simulink model "snap2_f_200msps_64i_4096c"  (R2019a)
settings: Solver=VariableStepDiscrete  StartTime=0.0  StopTime=10.0  RelTol=1e-3
undefined symbols (not defined in the file or in its folder): datetime, posixtime
libraries: xbsIndex_r4 x21354, casper_library_misc x297, casper_library_delays x19, xps_library x14, casper_library_sources x4
(part 34 of 217)

== system snap2_f_200msps_64i_4096c/noise/octal_mux4 ==
  n0 : Inport
  n1 : Inport  Port=2
  n2 : Inport  Port=3
  n3 : Inport  Port=4
  Delay{,1..7} (8 alike) : xbsIndex_r4/Delay  rst=off  infoeditControl=Selection of Reset will increase slice count due to use of real FFs and instead of SRLs  en=off  latency=1  reg_retiming=off  dbl_ovrd=off  block_type=delay
  Mux{,1..7} (8 alike) : xbsIndex_r4/Mux  inputs=4  en=off  latency=1  precision=Full  arith_type=Unsigned  n_bits=16  bin_pt=14  quantization=Truncate  overflow=Wrap  dbl_ovrd=off  block_type=mux
  Slice{,1..7} (8 alike) : xbsIndex_r4/Slice  nbits=2  boolean_output=off  mode=Lower Bit Location + Width  bit1=0  base1=MSB of Input  bit0=0  base0=LSB of Input  dbl_ovrd=off  block_type=slice
  bus_expand : Subsystem  AncestorBlock=casper_library_flow_control/bus_expand  mask(bus_expand){mode=divisions of equal size, outputNum=8, outputWidth=4, outputBinaryPt=0, outputArithmeticType=0, show_format=off, outputToWorkspace=off, variablePrefix=out, outputToModelAsWell=on}
      mask prompts: outputNum "Number of outputs:"; outputWidth "Output width:"; outputBinaryPt "Output binary point position:"; outputArithmeticType "Output arithmetic type (ufix=0, fix=1, bool=2):"; show_format "Print format string?"; outputToWorkspace "Output to workspace?"; variablePrefix "Variable name prefix:"; outputToModelAsWell "Output to model as well?"
      mask help:
      | Expands a 'bus' made using a bus_create or Xilinx
      | concat block.
      | The input will be divided into the specified number
      | of outputs with the specified arithmetic types.
      | Divisions are made from most significant bit.
      mask init: same as snap2_f_200msps_64i_4096c/autocorr/bus_expand
      settings: AttributesFormatString=8 outputs
      mask TypeOptions mode: divisions of equal size | divisions of arbitrary size
      mask Callback mode: bus_expand_callback();
      mask Callback outputWidth: bus_expand_callback();
      mask Callback outputToWorkspace: bus_expand_callback();
  sel : Subsystem  Tag=xps:sw_reg  AncestorBlock=xps_library/Memory/software_register  mask(swreg){io_dir=From Processor, io_delay=0, init_val=0, sample_period=1, names=reg, bitwidths=32, bin_pts=0, arith_types=0, sim_port=on, show_format=on, desc_str=|}
      mask desc_str=|
      | The lower 2 bits define the select signal for the
      | noise multiplexor. If this register has value ``v``, then noise generator
      | ``v`` is selected.
      mask prompts: io_dir "I/O direction"; io_delay "I/O delay"; init_val "Initial Value"; sample_period "Sample period"; names "Bitfield names [msb...lsb]"; bitwidths "Bitfield widths"; bin_pts "Bitfield binary pts"; arith_types "Bitfield types, ufix=0, fix=1, bool=2"; sim_port "Provide sim input/output?"; show_format "Print format string?"; desc_str "Description"
      mask help: A 32-bit software-accessible register. Can be divided into bitfields of varying widths and types using the fields in the block mask.
      mask init:
      | swreg_init(gcb)
      settings: AttributesFormatString=1input:uf32.0 = 32 bits
      mask TypeOptions io_dir: To Processor | From Processor
      mask Callback io_dir:
      | mask_enables = get_param(gcb, 'MaskEnables');
      | mask_names = get_param(gcb, 'MaskNames');
      | if strcmp(get_param(gcb, 'io_dir'), 'To Processor'),
      |     mask_enables{ismember(mask_names, 'sample_period')} = 'off';
      | else
      |     mask_enables{ismember(mask_names, 'sample_period')} = 'on';
      | end
      | set_param(gcb, 'MaskEnables', mask_enables);
      mask DialogControl ParameterTabVar0 Prompt: Setup
  out0 : Outport
  out1 : Outport  Port=2
  out2 : Outport  Port=3
  out3 : Outport  Port=4
  out4 : Outport  Port=5
  out5 : Outport  Port=6
  out6 : Outport  Port=7
  out7 : Outport  Port=8
  wires:
  Mux/1 -> out0/1
  n0/1 -> [noise0]
  n1/1 -> [noise1]
  n2/1 -> [noise2]
  n3/1 -> [noise3]
  [sel0] -> Delay/1
  [noise0] -> Mux/2
  [noise1] -> Mux/3
  [noise2] -> Mux/4
  [noise3] -> Mux/5
  [sel1] -> Delay1/1
  Mux1/1 -> out1/1
  sel/1(in_reg) -> bus_expand/1(bus_in)
  bus_expand/8(lsb_out1) -> Slice7/1
  bus_expand/7(out2) -> Slice6/1
  bus_expand/1(msb_out8) -> Slice/1
  bus_expand/2(out7) -> Slice1/1
  bus_expand/3(out6) -> Slice2/1
  bus_expand/4(out5) -> Slice3/1
  bus_expand/5(out4) -> Slice4/1
  bus_expand/6(out3) -> Slice5/1
  Mux3/1 -> out3/1
  [sel3] -> Delay3/1
  [sel2] -> Delay2/1
  Mux2/1 -> out2/1
  Mux6/1 -> out6/1
  [sel6] -> Delay5/1
  [sel7] -> Delay4/1
  Mux7/1 -> out7/1
  Mux5/1 -> out5/1
  [sel5] -> Delay6/1
  [sel4] -> Delay7/1
  Mux4/1 -> out4/1
  Slice/1 -> [sel7]
  Slice1/1 -> [sel6]
  Slice2/1 -> [sel5]
  Slice3/1 -> [sel4]
  Slice4/1 -> [sel3]
  Slice5/1 -> [sel2]
  Slice6/1 -> [sel1]
  Slice7/1 -> [sel0]
  [noise3] -> Mux1/5
  [noise2] -> Mux1/4
  [noise1] -> Mux1/3
  [noise0] -> Mux1/2
  [noise0] -> Mux2/2
  [noise1] -> Mux2/3
  [noise2] -> Mux2/4
  [noise3] -> Mux2/5
  [noise3] -> Mux3/5
  [noise2] -> Mux3/4
  [noise1] -> Mux3/3
  [noise0] -> Mux3/2
  [noise0] -> Mux4/2
  [noise1] -> Mux4/3
  [noise2] -> Mux4/4
  [noise3] -> Mux4/5
  [noise3] -> Mux5/5
  [noise2] -> Mux5/4
  [noise1] -> Mux5/3
  [noise0] -> Mux5/2
  [noise0] -> Mux6/2
  [noise1] -> Mux6/3
  [noise2] -> Mux6/4
  [noise3] -> Mux6/5
  [noise3] -> Mux7/5
  [noise2] -> Mux7/4
  [noise1] -> Mux7/3
  [noise0] -> Mux7/2
  Delay/1 -> Mux/1
  Delay1/1 -> Mux1/1
  Delay2/1 -> Mux2/1
  Delay3/1 -> Mux3/1
  Delay4/1 -> Mux7/1
  Delay5/1 -> Mux6/1
  Delay6/1 -> Mux5/1
  Delay7/1 -> Mux4/1

== system snap2_f_200msps_64i_4096c/noise/octal_mux5 ==
  n0 : Inport
  n1 : Inport  Port=2
  n2 : Inport  Port=3
  n3 : Inport  Port=4
  Delay{,1..7} (8 alike) : xbsIndex_r4/Delay  rst=off  infoeditControl=Selection of Reset will increase slice count due to use of real FFs and instead of SRLs  en=off  latency=1  reg_retiming=off  dbl_ovrd=off  block_type=delay
  Mux{,1..7} (8 alike) : xbsIndex_r4/Mux  inputs=4  en=off  latency=1  precision=Full  arith_type=Unsigned  n_bits=16  bin_pt=14  quantization=Truncate  overflow=Wrap  dbl_ovrd=off  block_type=mux
  Slice{,1..7} (8 alike) : xbsIndex_r4/Slice  nbits=2  boolean_output=off  mode=Lower Bit Location + Width  bit1=0  base1=MSB of Input  bit0=0  base0=LSB of Input  dbl_ovrd=off  block_type=slice
  bus_expand : Subsystem  AncestorBlock=casper_library_flow_control/bus_expand  mask(bus_expand){mode=divisions of equal size, outputNum=8, outputWidth=4, outputBinaryPt=0, outputArithmeticType=0, show_format=off, outputToWorkspace=off, variablePrefix=out, outputToModelAsWell=on}
      mask prompts: outputNum "Number of outputs:"; outputWidth "Output width:"; outputBinaryPt "Output binary point position:"; outputArithmeticType "Output arithmetic type (ufix=0, fix=1, bool=2):"; show_format "Print format string?"; outputToWorkspace "Output to workspace?"; variablePrefix "Variable name prefix:"; outputToModelAsWell "Output to model as well?"
      mask help:
      | Expands a 'bus' made using a bus_create or Xilinx
      | concat block.
      | The input will be divided into the specified number
      | of outputs with the specified arithmetic types.
      | Divisions are made from most significant bit.
      mask init: same as snap2_f_200msps_64i_4096c/autocorr/bus_expand
      settings: AttributesFormatString=8 outputs
      mask TypeOptions mode: divisions of equal size | divisions of arbitrary size
      mask Callback mode: bus_expand_callback();
      mask Callback outputWidth: bus_expand_callback();
      mask Callback outputToWorkspace: bus_expand_callback();
  sel : Subsystem  Tag=xps:sw_reg  AncestorBlock=xps_library/Memory/software_register  mask(swreg){io_dir=From Processor, io_delay=0, init_val=0, sample_period=1, names=reg, bitwidths=32, bin_pts=0, arith_types=0, sim_port=on, show_format=on, desc_str=|}
      mask desc_str=|
      | The lower 2 bits define the select signal for the
      | noise multiplexor. If this register has value ``v``, then noise generator
      | ``v`` is selected.
      mask prompts: io_dir "I/O direction"; io_delay "I/O delay"; init_val "Initial Value"; sample_period "Sample period"; names "Bitfield names [msb...lsb]"; bitwidths "Bitfield widths"; bin_pts "Bitfield binary pts"; arith_types "Bitfield types, ufix=0, fix=1, bool=2"; sim_port "Provide sim input/output?"; show_format "Print format string?"; desc_str "Description"
      mask help: A 32-bit software-accessible register. Can be divided into bitfields of varying widths and types using the fields in the block mask.
      mask init:
      | swreg_init(gcb)
      settings: AttributesFormatString=1input:uf32.0 = 32 bits
      mask TypeOptions io_dir: To Processor | From Processor
      mask Callback io_dir:
      | mask_enables = get_param(gcb, 'MaskEnables');
      | mask_names = get_param(gcb, 'MaskNames');
      | if strcmp(get_param(gcb, 'io_dir'), 'To Processor'),
      |     mask_enables{ismember(mask_names, 'sample_period')} = 'off';
      | else
      |     mask_enables{ismember(mask_names, 'sample_period')} = 'on';
      | end
      | set_param(gcb, 'MaskEnables', mask_enables);
      mask DialogControl ParameterTabVar0 Prompt: Setup
  out0 : Outport
  out1 : Outport  Port=2
  out2 : Outport  Port=3
  out3 : Outport  Port=4
  out4 : Outport  Port=5
  out5 : Outport  Port=6
  out6 : Outport  Port=7
  out7 : Outport  Port=8
  wires:
  Delay7/1 -> Mux4/1
  Delay6/1 -> Mux5/1
  Delay5/1 -> Mux6/1
  Delay4/1 -> Mux7/1
  Delay3/1 -> Mux3/1
  Delay2/1 -> Mux2/1
  Delay1/1 -> Mux1/1
  Delay/1 -> Mux/1
  [noise0] -> Mux7/2
  [noise1] -> Mux7/3
  [noise2] -> Mux7/4
  [noise3] -> Mux7/5
  [noise3] -> Mux6/5
  [noise2] -> Mux6/4
  [noise1] -> Mux6/3
  [noise0] -> Mux6/2
  [noise0] -> Mux5/2
  [noise1] -> Mux5/3
  [noise2] -> Mux5/4
  [noise3] -> Mux5/5
  [noise3] -> Mux4/5
  [noise2] -> Mux4/4
  [noise1] -> Mux4/3
  [noise0] -> Mux4/2
  [noise0] -> Mux3/2
  [noise1] -> Mux3/3
  [noise2] -> Mux3/4
  [noise3] -> Mux3/5
  [noise3] -> Mux2/5
  [noise2] -> Mux2/4
  [noise1] -> Mux2/3
  [noise0] -> Mux2/2
  [noise0] -> Mux1/2
  [noise1] -> Mux1/3
  [noise2] -> Mux1/4
  [noise3] -> Mux1/5
  Slice7/1 -> [sel0]
  Slice6/1 -> [sel1]
  Slice5/1 -> [sel2]
  Slice4/1 -> [sel3]
  Slice3/1 -> [sel4]
  Slice2/1 -> [sel5]
  Slice1/1 -> [sel6]
  Slice/1 -> [sel7]
  Mux4/1 -> out4/1
  [sel4] -> Delay7/1
  [sel5] -> Delay6/1
  Mux5/1 -> out5/1
  Mux7/1 -> out7/1
  [sel7] -> Delay4/1
  [sel6] -> Delay5/1
  Mux6/1 -> out6/1
  Mux2/1 -> out2/1
  [sel2] -> Delay2/1
  [sel3] -> Delay3/1
  Mux3/1 -> out3/1
  bus_expand/6(out3) -> Slice5/1
  bus_expand/5(out4) -> Slice4/1
  bus_expand/4(out5) -> Slice3/1
  bus_expand/3(out6) -> Slice2/1
  bus_expand/2(out7) -> Slice1/1
  bus_expand/1(msb_out8) -> Slice/1
  bus_expand/7(out2) -> Slice6/1
  bus_expand/8(lsb_out1) -> Slice7/1
  sel/1(in_reg) -> bus_expand/1(bus_in)
  Mux1/1 -> out1/1
  [sel1] -> Delay1/1
  [noise3] -> Mux/5
  [noise2] -> Mux/4
  [noise1] -> Mux/3
  [noise0] -> Mux/2
  [sel0] -> Delay/1
  n3/1 -> [noise3]
  n2/1 -> [noise2]
  n1/1 -> [noise1]
  n0/1 -> [noise0]
  Mux/1 -> out0/1

== system snap2_f_200msps_64i_4096c/noise/octal_mux6 ==
  n0 : Inport
  n1 : Inport  Port=2
  n2 : Inport  Port=3
  n3 : Inport  Port=4
  Delay{,1..7} (8 alike) : xbsIndex_r4/Delay  rst=off  infoeditControl=Selection of Reset will increase slice count due to use of real FFs and instead of SRLs  en=off  latency=1  reg_retiming=off  dbl_ovrd=off  block_type=delay
  Mux{,1..7} (8 alike) : xbsIndex_r4/Mux  inputs=4  en=off  latency=1  precision=Full  arith_type=Unsigned  n_bits=16  bin_pt=14  quantization=Truncate  overflow=Wrap  dbl_ovrd=off  block_type=mux
  Slice{,1..7} (8 alike) : xbsIndex_r4/Slice  nbits=2  boolean_output=off  mode=Lower Bit Location + Width  bit1=0  base1=MSB of Input  bit0=0  base0=LSB of Input  dbl_ovrd=off  block_type=slice
  bus_expand : Subsystem  AncestorBlock=casper_library_flow_control/bus_expand  mask(bus_expand){mode=divisions of equal size, outputNum=8, outputWidth=4, outputBinaryPt=0, outputArithmeticType=0, show_format=off, outputToWorkspace=off, variablePrefix=out, outputToModelAsWell=on}
      mask prompts: outputNum "Number of outputs:"; outputWidth "Output width:"; outputBinaryPt "Output binary point position:"; outputArithmeticType "Output arithmetic type (ufix=0, fix=1, bool=2):"; show_format "Print format string?"; outputToWorkspace "Output to workspace?"; variablePrefix "Variable name prefix:"; outputToModelAsWell "Output to model as well?"
      mask help:
      | Expands a 'bus' made using a bus_create or Xilinx
      | concat block.
      | The input will be divided into the specified number
      | of outputs with the specified arithmetic types.
      | Divisions are made from most significant bit.
      mask init: same as snap2_f_200msps_64i_4096c/autocorr/bus_expand
      settings: AttributesFormatString=8 outputs
      mask TypeOptions mode: divisions of equal size | divisions of arbitrary size
      mask Callback mode: bus_expand_callback();
      mask Callback outputWidth: bus_expand_callback();
      mask Callback outputToWorkspace: bus_expand_callback();
  sel : Subsystem  Tag=xps:sw_reg  AncestorBlock=xps_library/Memory/software_register  mask(swreg){io_dir=From Processor, io_delay=0, init_val=0, sample_period=1, names=reg, bitwidths=32, bin_pts=0, arith_types=0, sim_port=on, show_format=on, desc_str=|}
      mask desc_str=|
      | The lower 2 bits define the select signal for the
      | noise multiplexor. If this register has value ``v``, then noise generator
      | ``v`` is selected.
      mask prompts: io_dir "I/O direction"; io_delay "I/O delay"; init_val "Initial Value"; sample_period "Sample period"; names "Bitfield names [msb...lsb]"; bitwidths "Bitfield widths"; bin_pts "Bitfield binary pts"; arith_types "Bitfield types, ufix=0, fix=1, bool=2"; sim_port "Provide sim input/output?"; show_format "Print format string?"; desc_str "Description"
      mask help: A 32-bit software-accessible register. Can be divided into bitfields of varying widths and types using the fields in the block mask.
      mask init:
      | swreg_init(gcb)
      settings: AttributesFormatString=1input:uf32.0 = 32 bits
      mask TypeOptions io_dir: To Processor | From Processor
      mask Callback io_dir:
      | mask_enables = get_param(gcb, 'MaskEnables');
      | mask_names = get_param(gcb, 'MaskNames');
      | if strcmp(get_param(gcb, 'io_dir'), 'To Processor'),
      |     mask_enables{ismember(mask_names, 'sample_period')} = 'off';
      | else
      |     mask_enables{ismember(mask_names, 'sample_period')} = 'on';
      | end
      | set_param(gcb, 'MaskEnables', mask_enables);
      mask DialogControl ParameterTabVar0 Prompt: Setup
  out0 : Outport
  out1 : Outport  Port=2
  out2 : Outport  Port=3
  out3 : Outport  Port=4
  out4 : Outport  Port=5
  out5 : Outport  Port=6
  out6 : Outport  Port=7
  out7 : Outport  Port=8
  wires:
  Mux/1 -> out0/1
  n0/1 -> [noise0]
  n1/1 -> [noise1]
  n2/1 -> [noise2]
  n3/1 -> [noise3]
  [sel0] -> Delay/1
  [noise0] -> Mux/2
  [noise1] -> Mux/3
  [noise2] -> Mux/4
  [noise3] -> Mux/5
  [sel1] -> Delay1/1
  Mux1/1 -> out1/1
  sel/1(in_reg) -> bus_expand/1(bus_in)
  bus_expand/8(lsb_out1) -> Slice7/1
  bus_expand/7(out2) -> Slice6/1
  bus_expand/1(msb_out8) -> Slice/1
  bus_expand/2(out7) -> Slice1/1
  bus_expand/3(out6) -> Slice2/1
  bus_expand/4(out5) -> Slice3/1
  bus_expand/5(out4) -> Slice4/1
  bus_expand/6(out3) -> Slice5/1
  Mux3/1 -> out3/1
  [sel3] -> Delay3/1
  [sel2] -> Delay2/1
  Mux2/1 -> out2/1
  Mux6/1 -> out6/1
  [sel6] -> Delay5/1
  [sel7] -> Delay4/1
  Mux7/1 -> out7/1
  Mux5/1 -> out5/1
  [sel5] -> Delay6/1
  [sel4] -> Delay7/1
  Mux4/1 -> out4/1
  Slice/1 -> [sel7]
  Slice1/1 -> [sel6]
  Slice2/1 -> [sel5]
  Slice3/1 -> [sel4]
  Slice4/1 -> [sel3]
  Slice5/1 -> [sel2]
  Slice6/1 -> [sel1]
  Slice7/1 -> [sel0]
  [noise3] -> Mux1/5
  [noise2] -> Mux1/4
  [noise1] -> Mux1/3
  [noise0] -> Mux1/2
  [noise0] -> Mux2/2
  [noise1] -> Mux2/3
  [noise2] -> Mux2/4
  [noise3] -> Mux2/5
  [noise3] -> Mux3/5
  [noise2] -> Mux3/4
  [noise1] -> Mux3/3
  [noise0] -> Mux3/2
  [noise0] -> Mux4/2
  [noise1] -> Mux4/3
  [noise2] -> Mux4/4
  [noise3] -> Mux4/5
  [noise3] -> Mux5/5
  [noise2] -> Mux5/4
  [noise1] -> Mux5/3
  [noise0] -> Mux5/2
  [noise0] -> Mux6/2
  [noise1] -> Mux6/3
  [noise2] -> Mux6/4
  [noise3] -> Mux6/5
  [noise3] -> Mux7/5
  [noise2] -> Mux7/4
  [noise1] -> Mux7/3
  [noise0] -> Mux7/2
  Delay/1 -> Mux/1
  Delay1/1 -> Mux1/1
  Delay2/1 -> Mux2/1
  Delay3/1 -> Mux3/1
  Delay4/1 -> Mux7/1
  Delay5/1 -> Mux6/1
  Delay6/1 -> Mux5/1
  Delay7/1 -> Mux4/1

== system snap2_f_200msps_64i_4096c/noise/octal_mux7 ==
  n0 : Inport
  n1 : Inport  Port=2
  n2 : Inport  Port=3
  n3 : Inport  Port=4
  Delay{,1..7} (8 alike) : xbsIndex_r4/Delay  rst=off  infoeditControl=Selection of Reset will increase slice count due to use of real FFs and instead of SRLs  en=off  latency=1  reg_retiming=off  dbl_ovrd=off  block_type=delay
  Mux{,1..7} (8 alike) : xbsIndex_r4/Mux  inputs=4  en=off  latency=1  precision=Full  arith_type=Unsigned  n_bits=16  bin_pt=14  quantization=Truncate  overflow=Wrap  dbl_ovrd=off  block_type=mux
  Slice{,1..7} (8 alike) : xbsIndex_r4/Slice  nbits=2  boolean_output=off  mode=Lower Bit Location + Width  bit1=0  base1=MSB of Input  bit0=0  base0=LSB of Input  dbl_ovrd=off  block_type=slice
  bus_expand : Subsystem  AncestorBlock=casper_library_flow_control/bus_expand  mask(bus_expand){mode=divisions of equal size, outputNum=8, outputWidth=4, outputBinaryPt=0, outputArithmeticType=0, show_format=off, outputToWorkspace=off, variablePrefix=out, outputToModelAsWell=on}
      mask prompts: outputNum "Number of outputs:"; outputWidth "Output width:"; outputBinaryPt "Output binary point position:"; outputArithmeticType "Output arithmetic type (ufix=0, fix=1, bool=2):"; show_format "Print format string?"; outputToWorkspace "Output to workspace?"; variablePrefix "Variable name prefix:"; outputToModelAsWell "Output to model as well?"
      mask help:
      | Expands a 'bus' made using a bus_create or Xilinx
      | concat block.
      | The input will be divided into the specified number
      | of outputs with the specified arithmetic types.
      | Divisions are made from most significant bit.
      mask init: same as snap2_f_200msps_64i_4096c/autocorr/bus_expand
      settings: AttributesFormatString=8 outputs
      mask TypeOptions mode: divisions of equal size | divisions of arbitrary size
      mask Callback mode: bus_expand_callback();
      mask Callback outputWidth: bus_expand_callback();
      mask Callback outputToWorkspace: bus_expand_callback();
  sel : Subsystem  Tag=xps:sw_reg  AncestorBlock=xps_library/Memory/software_register  mask(swreg){io_dir=From Processor, io_delay=0, init_val=0, sample_period=1, names=reg, bitwidths=32, bin_pts=0, arith_types=0, sim_port=on, show_format=on, desc_str=|}
      mask desc_str=|
      | The lower 2 bits define the select signal for the
      | noise multiplexor. If this register has value ``v``, then noise generator
      | ``v`` is selected.
      mask prompts: io_dir "I/O direction"; io_delay "I/O delay"; init_val "Initial Value"; sample_period "Sample period"; names "Bitfield names [msb...lsb]"; bitwidths "Bitfield widths"; bin_pts "Bitfield binary pts"; arith_types "Bitfield types, ufix=0, fix=1, bool=2"; sim_port "Provide sim input/output?"; show_format "Print format string?"; desc_str "Description"
      mask help: A 32-bit software-accessible register. Can be divided into bitfields of varying widths and types using the fields in the block mask.
      mask init:
      | swreg_init(gcb)
      settings: AttributesFormatString=1input:uf32.0 = 32 bits
      mask TypeOptions io_dir: To Processor | From Processor
      mask Callback io_dir:
      | mask_enables = get_param(gcb, 'MaskEnables');
      | mask_names = get_param(gcb, 'MaskNames');
      | if strcmp(get_param(gcb, 'io_dir'), 'To Processor'),
      |     mask_enables{ismember(mask_names, 'sample_period')} = 'off';
      | else
      |     mask_enables{ismember(mask_names, 'sample_period')} = 'on';
      | end
      | set_param(gcb, 'MaskEnables', mask_enables);
      mask DialogControl ParameterTabVar0 Prompt: Setup
  out0 : Outport
  out1 : Outport  Port=2
  out2 : Outport  Port=3
  out3 : Outport  Port=4
  out4 : Outport  Port=5
  out5 : Outport  Port=6
  out6 : Outport  Port=7
  out7 : Outport  Port=8
  wires:
  Delay7/1 -> Mux4/1
  Delay6/1 -> Mux5/1
  Delay5/1 -> Mux6/1
  Delay4/1 -> Mux7/1
  Delay3/1 -> Mux3/1
  Delay2/1 -> Mux2/1
  Delay1/1 -> Mux1/1
  Delay/1 -> Mux/1
  [noise0] -> Mux7/2
  [noise1] -> Mux7/3
  [noise2] -> Mux7/4
  [noise3] -> Mux7/5
  [noise3] -> Mux6/5
  [noise2] -> Mux6/4
  [noise1] -> Mux6/3
  [noise0] -> Mux6/2
  [noise0] -> Mux5/2
  [noise1] -> Mux5/3
  [noise2] -> Mux5/4
  [noise3] -> Mux5/5
  [noise3] -> Mux4/5
  [noise2] -> Mux4/4
  [noise1] -> Mux4/3
  [noise0] -> Mux4/2
  [noise0] -> Mux3/2
  [noise1] -> Mux3/3
  [noise2] -> Mux3/4
  [noise3] -> Mux3/5
  [noise3] -> Mux2/5
  [noise2] -> Mux2/4
  [noise1] -> Mux2/3
  [noise0] -> Mux2/2
  [noise0] -> Mux1/2
  [noise1] -> Mux1/3
  [noise2] -> Mux1/4
  [noise3] -> Mux1/5
  Slice7/1 -> [sel0]
  Slice6/1 -> [sel1]
  Slice5/1 -> [sel2]
  Slice4/1 -> [sel3]
  Slice3/1 -> [sel4]
  Slice2/1 -> [sel5]
  Slice1/1 -> [sel6]
  Slice/1 -> [sel7]
  Mux4/1 -> out4/1
  [sel4] -> Delay7/1
  [sel5] -> Delay6/1
  Mux5/1 -> out5/1
  Mux7/1 -> out7/1
  [sel7] -> Delay4/1
  [sel6] -> Delay5/1
  Mux6/1 -> out6/1
  Mux2/1 -> out2/1
  [sel2] -> Delay2/1
  [sel3] -> Delay3/1
  Mux3/1 -> out3/1
  bus_expand/6(out3) -> Slice5/1
  bus_expand/5(out4) -> Slice4/1
  bus_expand/4(out5) -> Slice3/1
  bus_expand/3(out6) -> Slice2/1
  bus_expand/2(out7) -> Slice1/1
  bus_expand/1(msb_out8) -> Slice/1
  bus_expand/7(out2) -> Slice6/1
  bus_expand/8(lsb_out1) -> Slice7/1
  sel/1(in_reg) -> bus_expand/1(bus_in)
  Mux1/1 -> out1/1
  [sel1] -> Delay1/1
  [noise3] -> Mux/5
  [noise2] -> Mux/4
  [noise1] -> Mux/3
  [noise0] -> Mux/2
  [sel0] -> Delay/1
  n3/1 -> [noise3]
  n2/1 -> [noise2]
  n1/1 -> [noise1]
  n0/1 -> [noise0]
  Mux/1 -> out0/1

== system snap2_f_200msps_64i_4096c/noise/octal_mux8 ==
  n0 : Inport
  n1 : Inport  Port=2
  n2 : Inport  Port=3
  n3 : Inport  Port=4
  n4 : Inport  Port=5
  n5 : Inport  Port=6
  n6 : Inport  Port=7
  n7 : Inport  Port=8
  Mux{,1..7} (8 alike) : xbsIndex_r4/Mux  inputs=8  en=off  latency=1  precision=Full  arith_type=Unsigned  n_bits=16  bin_pt=14  quantization=Truncate  overflow=Wrap  dbl_ovrd=off  block_type=mux
  Slice{,1..7} (8 alike) : xbsIndex_r4/Slice  nbits=3  boolean_output=off  mode=Lower Bit Location + Width  bit1=0  base1=MSB of Input  bit0=0  base0=LSB of Input  dbl_ovrd=off  block_type=slice
  bus_expand : Subsystem  AncestorBlock=casper_library_flow_control/bus_expand  mask(bus_expand){mode=divisions of equal size, outputNum=8, outputWidth=4, outputBinaryPt=0, outputArithmeticType=0, show_format=off, outputToWorkspace=off, variablePrefix=out, outputToModelAsWell=on}
      mask prompts: outputNum "Number of outputs:"; outputWidth "Output width:"; outputBinaryPt "Output binary point position:"; outputArithmeticType "Output arithmetic type (ufix=0, fix=1, bool=2):"; show_format "Print format string?"; outputToWorkspace "Output to workspace?"; variablePrefix "Variable name prefix:"; outputToModelAsWell "Output to model as well?"
      mask help:
      | Expands a 'bus' made using a bus_create or Xilinx
      | concat block.
      | The input will be divided into the specified number
      | of outputs with the specified arithmetic types.
      | Divisions are made from most significant bit.
      mask init: same as snap2_f_200msps_64i_4096c/autocorr/bus_expand
      settings: AttributesFormatString=8 outputs
      mask TypeOptions mode: divisions of equal size | divisions of arbitrary size
      mask Callback mode: bus_expand_callback();
      mask Callback outputWidth: bus_expand_callback();
      mask Callback outputToWorkspace: bus_expand_callback();
  sel : Subsystem  Tag=xps:sw_reg  AncestorBlock=xps_library/Memory/software_register  mask(swreg){io_dir=From Processor, io_delay=0, init_val=0, sample_period=1, names=reg, bitwidths=32, bin_pts=0, arith_types=0, sim_port=on, show_format=on, desc_str=|}
      mask desc_str=|
      | The lower 2 bits define the select signal for the
      | noise multiplexor. If this register has value ``v``, then noise generator
      | ``v`` is selected.
      mask prompts: io_dir "I/O direction"; io_delay "I/O delay"; init_val "Initial Value"; sample_period "Sample period"; names "Bitfield names [msb...lsb]"; bitwidths "Bitfield widths"; bin_pts "Bitfield binary pts"; arith_types "Bitfield types, ufix=0, fix=1, bool=2"; sim_port "Provide sim input/output?"; show_format "Print format string?"; desc_str "Description"
      mask help: A 32-bit software-accessible register. Can be divided into bitfields of varying widths and types using the fields in the block mask.
      mask init:
      | swreg_init(gcb)
      settings: AttributesFormatString=1input:uf32.0 = 32 bits
      mask TypeOptions io_dir: To Processor | From Processor
      mask Callback io_dir:
      | mask_enables = get_param(gcb, 'MaskEnables');
      | mask_names = get_param(gcb, 'MaskNames');
      | if strcmp(get_param(gcb, 'io_dir'), 'To Processor'),
      |     mask_enables{ismember(mask_names, 'sample_period')} = 'off';
      | else
      |     mask_enables{ismember(mask_names, 'sample_period')} = 'on';
      | end
      | set_param(gcb, 'MaskEnables', mask_enables);
      mask DialogControl ParameterTabVar0 Prompt: Setup
  out0 : Outport
  out1 : Outport  Port=2
  out2 : Outport  Port=3
  out3 : Outport  Port=4
  out4 : Outport  Port=5
  out5 : Outport  Port=6
  out6 : Outport  Port=7
  out7 : Outport  Port=8
  wires:
  Slice7/1 -> [sel0]
  Slice6/1 -> [sel1]
  Slice5/1 -> [sel2]
  Slice4/1 -> [sel3]
  Slice3/1 -> [sel4]
  Slice2/1 -> [sel5]
  Slice1/1 -> [sel6]
  Slice/1 -> [sel7]
  Mux4/1 -> out4/1
  [sel4] -> Mux4/1
  [noise0] -> Mux4/2
  [noise1] -> Mux4/3
  [noise2] -> Mux4/4
  [noise3] -> Mux4/5
  [noise4] -> Mux4/6
  [noise5] -> Mux4/7
  [noise6] -> Mux4/8
  [noise7] -> Mux4/9
  [noise7] -> Mux5/9
  [noise6] -> Mux5/8
  [noise5] -> Mux5/7
  [noise4] -> Mux5/6
  [noise3] -> Mux5/5
  [noise2] -> Mux5/4
  [noise1] -> Mux5/3
  [noise0] -> Mux5/2
  [sel5] -> Mux5/1
  Mux5/1 -> out5/1
  Mux7/1 -> out7/1
  [sel7] -> Mux7/1
  [noise0] -> Mux7/2
  [noise1] -> Mux7/3
  [noise2] -> Mux7/4
  [noise3] -> Mux7/5
  [noise4] -> Mux7/6
  [noise5] -> Mux7/7
  [noise6] -> Mux7/8
  [noise7] -> Mux7/9
  [noise7] -> Mux6/9
  [noise6] -> Mux6/8
  [noise5] -> Mux6/7
  [noise4] -> Mux6/6
  [noise3] -> Mux6/5
  [noise2] -> Mux6/4
  [noise1] -> Mux6/3
  [noise0] -> Mux6/2
  [sel6] -> Mux6/1
  Mux6/1 -> out6/1
  Mux2/1 -> out2/1
  [sel2] -> Mux2/1
  [noise0] -> Mux2/2
  [noise1] -> Mux2/3
  [noise2] -> Mux2/4
  [noise3] -> Mux2/5
  [noise4] -> Mux2/6
  [noise5] -> Mux2/7
  [noise6] -> Mux2/8
  [noise7] -> Mux2/9
  [noise7] -> Mux3/9
  [noise6] -> Mux3/8
  [noise5] -> Mux3/7
  [noise4] -> Mux3/6
  [noise3] -> Mux3/5
  [noise2] -> Mux3/4
  [noise1] -> Mux3/3
  [noise0] -> Mux3/2
  [sel3] -> Mux3/1
  Mux3/1 -> out3/1
  bus_expand/6(out3) -> Slice5/1
  bus_expand/5(out4) -> Slice4/1
  bus_expand/4(out5) -> Slice3/1
  bus_expand/3(out6) -> Slice2/1
  bus_expand/2(out7) -> Slice1/1
  bus_expand/1(msb_out8) -> Slice/1
  bus_expand/7(out2) -> Slice6/1
  bus_expand/8(lsb_out1) -> Slice7/1
  sel/1(in_reg) -> bus_expand/1(bus_in)
  Mux1/1 -> out1/1
  [sel1] -> Mux1/1
  [noise0] -> Mux1/2
  [noise1] -> Mux1/3
  [noise2] -> Mux1/4
  [noise3] -> Mux1/5
  [noise4] -> Mux1/6
  [noise5] -> Mux1/7
  [noise6] -> Mux1/8
  [noise7] -> Mux1/9
  [noise7] -> Mux/9
  [noise6] -> Mux/8
  [noise5] -> Mux/7
  [noise4] -> Mux/6
  [noise3] -> Mux/5
  [noise2] -> Mux/4
  [noise1] -> Mux/3
  [noise0] -> Mux/2
  [sel0] -> Mux/1
  n7/1 -> [noise7]
  n6/1 -> [noise6]
  n5/1 -> [noise5]
  n4/1 -> [noise4]
  n3/1 -> [noise3]
  n2/1 -> [noise2]
  n1/1 -> [noise1]
  n0/1 -> [noise0]
  Mux/1 -> out0/1

== system snap2_f_200msps_64i_4096c/noise/seeds0 ==
  sim_1 : Inport
  convert1_1 : DataTypeConversion  OutDataTypeStr=fixdt('ufix32_En0')  LockScale=on
  convert2_1 : DataTypeConversion  OutDataTypeStr=fixdt('ufix32_En0')  ConvertRealWorld=Stored Integer (SI)  LockScale=on
  gain_1 : Gain
  io_delay : xbsIndex_r4/Delay  rst=off  infoeditControl=Selection of Reset will increase slice count due to use of real FFs and instead of SRLs  en=off  latency=0  reg_retiming=on  dbl_ovrd=off  block_type=delay
  reint1 : xbsIndex_r4/Reinterpret  force_arith_type=on  arith_type=Unsigned  force_bin_pt=on  bin_pt=0  block_type=reinterpret
  slice_reg : xbsIndex_r4/Slice  nbits=32  boolean_output=off  mode=Lower Bit Location + Width  bit1=0  base1=MSB of Input  bit0=0  base0=LSB of Input  dbl_ovrd=off  block_type=slice
  snap2_f_200msps_64i_4096c_noise_seeds0_user_data_out : xbsIndex_r4/Gateway In  gui_display_data_type=Fixed-point  arith_type=Unsigned  n_bits=32  bin_pt=0  preci_type=Single  exp_width=8  frac_width=24  rows=1  columns=1  quantization="Round  (unbiased: +/- Inf)"  overflow=Saturate  period=1  UseAsADC=off  ADCChannel='1'  interface=None  automatic_assignment=on  address_offset=hex2dec('00')  intf_name=''  intf_description=''  default_value=0  timing_constraint=None  locs_specified=off  LOCs={}  io_standard={}  inherit_from_input=off  hdl_port=on  dbl_ovrd=off  block_type=gatewayin
  in_reg : Outport
  wires:
  snap2_f_200msps_64i_4096c_noise_seeds0_user_data_out/1 -> io_delay/1
  sim_1/1 -> convert1_1/1
  convert1_1/1 -> convert2_1/1
  convert2_1/1 -> gain_1/1
  gain_1/1 -> snap2_f_200msps_64i_4096c_noise_seeds0_user_data_out/1
  io_delay/1 -> slice_reg/1
  slice_reg/1 -> reint1/1
  reint1/1 -> in_reg/1
